simulink model "gm_hdl_dut_bch_encoder"  (R2020b)
settings: Solver=FixedStepDiscrete  StartTime=0.0  StopTime=1  RelTol=1e-3
undefined symbols (not defined in the file): message
settings Model: Creator=wardo  LastModifiedBy=wardo
settings DataIOCC: LimitDataPoints=on  SaveOutput=off  SaveTime=off
settings OptimizationCC: BlockReduction=off  ConditionallyExecuteInputs=off  DefaultParameterBehavior=Inlined  LifeSpan=inf
settings DebuggingCC: AlgebraicLoopMsg=error  InheritedTsInSrcMsg=none  SingleTaskRateTransMsg=error  AllowSymbolicDim=off  StrictBusMsg=ErrorOnBusTreatedAsVector  SFUnexpectedBacktrackingDiag=warning  SFNoUnconditionalDefaultTransitionDiag=warning  SFExecutionAtInitializationDiag=none  ArithmeticOperatorsInVariantConditions=warning
settings HardwareCC: ProdBitPerPointer=32  ProdBitPerSizeT=32  ProdBitPerPtrDiffT=32  ProdLargestAtomicFloat=None  ProdIntDivRoundTo=Undefined  ProdEndianess=Unspecified  ProdWordSize=32  ProdHWDeviceType=ASIC/FPGA->ASIC/FPGA  ProdEqTarget=off
settings SFSimCC: SimUseLocalCustomCode=off  CustomCodeUndefinedFunction=UseInterfaceOnly
settings RTWCC: RTWUseLocalCustomCode=off
settings CodeAppCC: StateflowObjectComments=on
settings GRTTargetCC: TargetLangStandard=C89/C90 (ANSI)
settings ConfigComp: CovScope=ReferencedModels  CovMetricSettings=dw  CovSaveCumulativeToWorkspaceVar=on  CovSaveSingleToWorkspaceVar=on  CovExternalEMLEnable=off  CovSFcnEnable=off

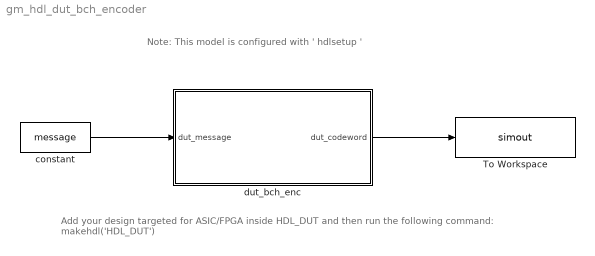
== system gm_hdl_dut_bch_encoder ==
  note: Add your design targeted for ASIC/FPGA inside HDL_DUT and then run the following command:
      | makehdl('HDL_DUT')
  note: Note: This model is configured with ' hdlsetup '
  To Workspace : ToWorkspace  VariableName=simout  SaveFormat=Timeseries  SampleTime=-1
  constant : Constant  Value=message  SampleTime=-1
  dut_bch_enc : Subsystem
  wires:
  dut_bch_enc/1(dut_codeword) -> To Workspace/1
  constant/1 -> dut_bch_enc/1(dut_message)

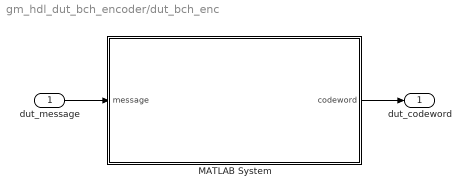
== system gm_hdl_dut_bch_encoder/dut_bch_enc ==
  dut_message : Inport  OutDataTypeStr=boolean  PortDimensions=[48408]  SampleTime=0.02
  MATLAB System : Subsystem
  dut_codeword : Outport  VectorParamsAs1DForOutWhenUnconnected=off
  wires:
  dut_message/1 -> MATLAB System/1(message)
  MATLAB System/1(codeword) -> dut_codeword/1

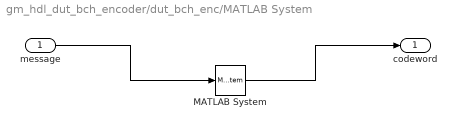
== system gm_hdl_dut_bch_encoder/dut_bch_enc/MATLAB System ==
  message : Inport  OutDataTypeStr=boolean  PortDimensions=[48408]  SampleTime=0.02
  MATLAB System : MATLABSystem  System=BCHEncoder  SimulateUsing=Code generation
      mask Type: BCHEncoder
      mask Display:
      | disp('BCHEncoder');
      | port_label('input',1,'message');
      | port_label('output',1,'codeword');
  codeword : Outport
  wires:
  message/1 -> MATLAB System/1
  MATLAB System/1 -> codeword/1
